simulink model "sampleModel354"  (R2021b)
settings: Solver=VariableStepAuto  StartTime=0.0  StopTime=10.0  RelTol=1e-3
libraries: simulink x2, slpidlib x1
settings Model: Creator=user  LastModifiedBy=user

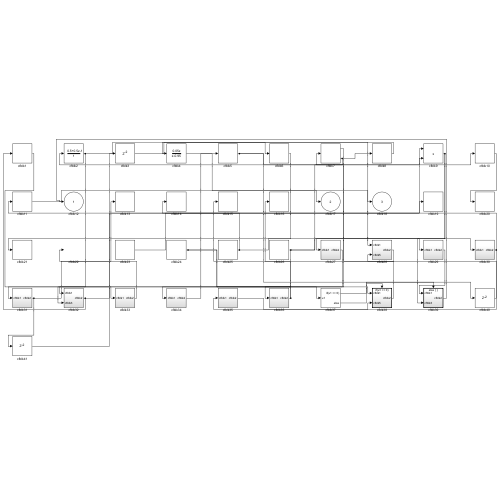
[thumbnail: Simulink's stored preview of the top-level diagram]
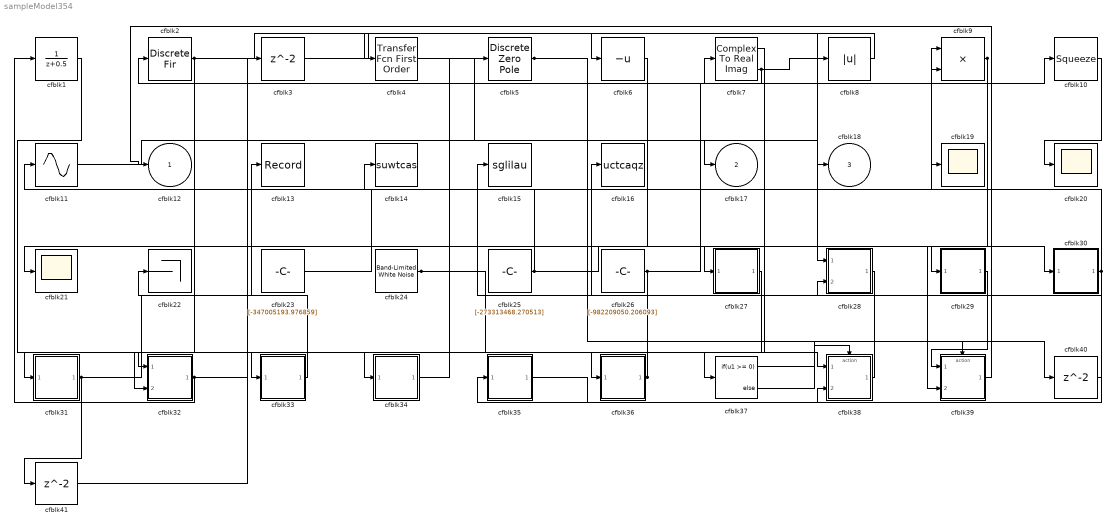
== system sampleModel354 ==
  cfblk1 : DiscreteTransferFcn  SampleTime=1
  cfblk10 : Squeeze
  cfblk11 : Sin  TimeSource=Use external signal  SampleTime=0
  cfblk13 : Record  FileSettingsInternal="{\"entries\":[{\"content\":{\"excelSettings\":{\"content\":{},\"type\":\"Streamout.ExcelSettings\"}},\"type\":\"Streamout.FileSettingStorage\",\"uuid\":\"651ccca9-41b0-448b-87a9-5c5838d69a5d\"}],\"packageUris\":[\"http://schema.mathworks.com/mf0/streamout_blocks/R2020a\"],\"version\":\"1.0\"}"  SignalsInternal="{\"entries\":[{\"content\":{\"signals\":[{\"content\":{\"blockPath\":[\"sampleModel354/cfblk13\"],\"channel\":[],\"dimensions\":[1],\"domain\":\"sampleModel354/cfblk13\",\"lineColor\":\"#b746ff\",\"plots\":[1],\"port\":1,\"sid\":[\"\"],\"signalID\":14731,\"signalName\":\"cfblk31\"},\"type\":\"RecordBlkView.Signal\",\"uuid\":\"0d68e5df-fecc-40d7-916a-77594ce0a885\"}]},\"type\":\"RecordBlkView.InputSignals\",\"uuid\":\"2bd33199-b1ec-44f2-9605-e6013ce188e2\"}],\"packageUris\":[\"http://schema.mathworks.com/mf0/streamout_blocks/R2020a\"],\"version\":\"1.0\"}"  VisualizationBindings="{\"sparklinesplugin\":{\"info\":[{\"bindingParametersList\":[],\"subplotID\":1}]}}"
  cfblk14 : ToWorkspace  VariableName=suwtcas  SaveFormat=Timeseries  SampleTime=-1
  cfblk15 : ToWorkspace  VariableName=sglilau  SaveFormat=Timeseries  SampleTime=-1
  cfblk16 : ToWorkspace  VariableName=uctcaqz  SaveFormat=Timeseries  SampleTime=-1
  cfblk19 : Scope
  cfblk2 : DiscreteFir  SampleTime=1
  cfblk20 : Scope
  cfblk21 : Scope
  cfblk22 : Terminator
  cfblk23 : Constant  Value=[-347005193.976859]  SampleTime=1
  cfblk24 : simulink/Sources/Band-Limited White Noise  Cov=[1107350414.755051]  Ts=0.1  seed=[9554781753.000000]
  cfblk25 : Constant  Value=[-273313468.270513]  SampleTime=1
  cfblk26 : Constant  Value=[-982209050.206093]  SampleTime=1
  cfblk27 : Subsystem
  cfblk28 : Subsystem
  cfblk29 : Subsystem
  cfblk3 : Delay  SampleTime=1
  cfblk30 : Subsystem
  cfblk31 : Subsystem
  cfblk32 : Subsystem
  cfblk33 : Subsystem
  cfblk34 : Subsystem
  cfblk35 : Subsystem
  cfblk36 : Subsystem
  cfblk37 : If  IfExpression=u1 >= 0  SampleTime=1
  cfblk38 : Subsystem  TreatAsAtomicUnit=on
  cfblk39 : Subsystem  TreatAsAtomicUnit=on
  cfblk4 : simulink/Discrete/Transfer Fcn First Order  PoleZ=0.95  ICPrevOutput=0.0  DoSatur=off
  cfblk40 : Delay  SampleTime=1
  cfblk41 : Delay  SampleTime=1
  cfblk5 : DiscreteZeroPole  Poles=[0 0.5]  Gain=1
  cfblk6 : UnaryMinus
  cfblk7 : ComplexToRealImag
  cfblk8 : Abs
  cfblk9 : Product
  cfblk12 : Outport
  cfblk17 : Outport  Port=2
  cfblk18 : Outport  Port=3
  wires:
  cfblk34/1(cfblk2) -> cfblk5/1
  cfblk3/1 -> cfblk28/1(cfblk1)
  cfblk27/1(cfblk2) -> cfblk36/1(cfblk1)
  cfblk28/1(cfblk2) -> cfblk7/1
  cfblk6/1 -> cfblk21/1
  cfblk29/1(cfblk2) -> cfblk39/1(cfblk1)
  cfblk1/1 -> cfblk33/1(cfblk1)
  cfblk38/1(cfblk2) -> cfblk16/1
  cfblk5/1 -> cfblk9/2, cfblk40/1
  cfblk9/1 -> cfblk27/1(cfblk1), cfblk39/2(cfblk3)
  cfblk7/1 -> cfblk34/1(cfblk1)
  cfblk10/1 -> cfblk20/1
  cfblk7/2 -> cfblk2/1, cfblk8/1
  cfblk33/1(cfblk2) -> cfblk22/1
  cfblk4/1 -> cfblk17/1
  cfblk24/1 -> cfblk38/1(cfblk1), cfblk37/1
  cfblk30/1(cfblk2) -> cfblk35/1(cfblk1), cfblk14/1
  cfblk2/1 -> cfblk6/1, cfblk32/1(cfblk1)
  cfblk11/1 -> cfblk18/1
  cfblk39/1(cfblk2) -> cfblk12/1
  cfblk23/1 -> cfblk9/1
  cfblk36/1(cfblk2) -> cfblk15/1, cfblk31/1(cfblk1)
  cfblk31/1(cfblk2) -> cfblk13/1, cfblk41/1
  cfblk8/1 -> cfblk4/1
  cfblk25/1 -> cfblk11/1, cfblk29/1(cfblk1)
  cfblk26/1 -> cfblk10/1, cfblk32/2(cfblk3), cfblk30/1(cfblk1)
  cfblk35/1(cfblk2) -> cfblk38/2(cfblk5)
  cfblk32/1(cfblk2) -> cfblk1/1, cfblk19/1
  cfblk37/1 -> cfblk38/Action
  cfblk37/2 -> cfblk39/Action
  cfblk40/1 -> cfblk28/2(cfblk5)
  cfblk41/1 -> cfblk3/1

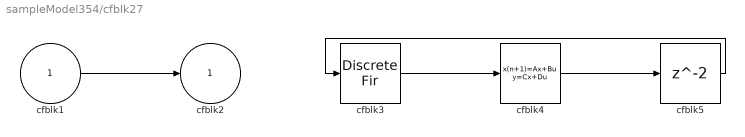
== system sampleModel354/cfblk27 ==
  cfblk1 : Inport
  cfblk3 : DiscreteFir  SampleTime=1
  cfblk4 : DiscreteStateSpace
  cfblk5 : Delay  SampleTime=1
  cfblk2 : Outport
  wires:
  cfblk1/1 -> cfblk2/1
  cfblk3/1 -> cfblk4/1
  cfblk4/1 -> cfblk5/1
  cfblk5/1 -> cfblk3/1

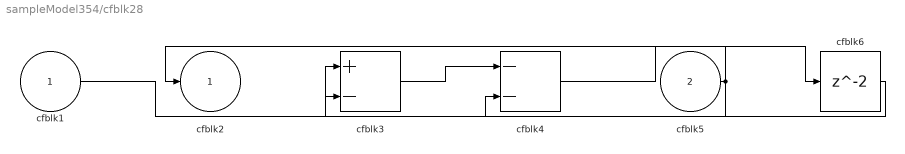
== system sampleModel354/cfblk28 ==
  cfblk1 : Inport
  cfblk5 : Inport  Port=2
  cfblk3 : Sum  Inputs=+-
  cfblk4 : Sum  Inputs=--
  cfblk6 : Delay  SampleTime=1
  cfblk2 : Outport
  wires:
  cfblk5/1 -> cfblk2/1, cfblk4/2
  cfblk1/1 -> cfblk3/1
  cfblk3/1 -> cfblk4/1
  cfblk4/1 -> cfblk6/1
  cfblk6/1 -> cfblk3/2

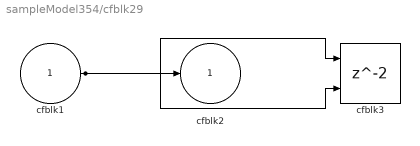
== system sampleModel354/cfblk29 ==
  cfblk1 : Inport
  cfblk3 : Delay  ShowEnablePort=on  SampleTime=1
      settings: InputPortMap=u0,e6
  cfblk2 : Outport
  wires:
  cfblk1/1 -> cfblk2/1, cfblk3/1, cfblk3/2

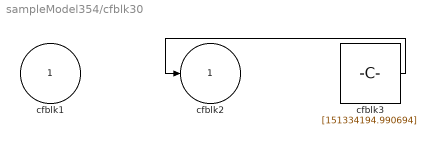
== system sampleModel354/cfblk30 ==
  cfblk1 : Inport
  cfblk3 : Constant  Value=[151334194.990694]  SampleTime=1
  cfblk2 : Outport
  wires:
  cfblk3/1 -> cfblk2/1

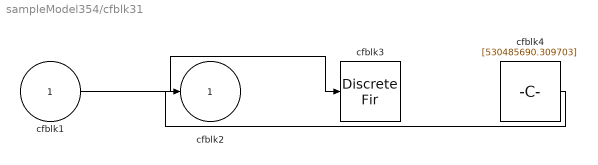
== system sampleModel354/cfblk31 ==
  cfblk1 : Inport
  cfblk3 : DiscreteFir  SampleTime=1
  cfblk4 : Constant  Value=[530485690.309703]  SampleTime=1
  cfblk2 : Outport
  wires:
  cfblk1/1 -> cfblk3/1
  cfblk4/1 -> cfblk2/1

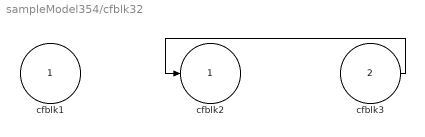
== system sampleModel354/cfblk32 ==
  cfblk1 : Inport
  cfblk3 : Inport  Port=2
  cfblk2 : Outport
  wires:
  cfblk3/1 -> cfblk2/1

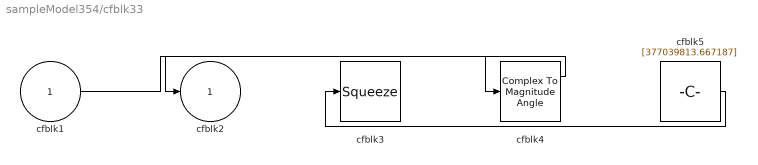
== system sampleModel354/cfblk33 ==
  cfblk1 : Inport
  cfblk3 : Squeeze
  cfblk4 : ComplexToMagnitudeAngle
  cfblk5 : Constant  Value=[377039813.667187]  SampleTime=1
  cfblk2 : Outport
  wires:
  cfblk4/1 -> cfblk2/1
  cfblk5/1 -> cfblk3/1
  cfblk1/1 -> cfblk4/1

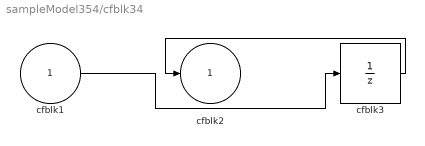
== system sampleModel354/cfblk34 ==
  cfblk1 : Inport
  cfblk3 : UnitDelay  HasFrameUpgradeWarning=on
  cfblk2 : Outport
  wires:
  cfblk3/1 -> cfblk2/1
  cfblk1/1 -> cfblk3/1

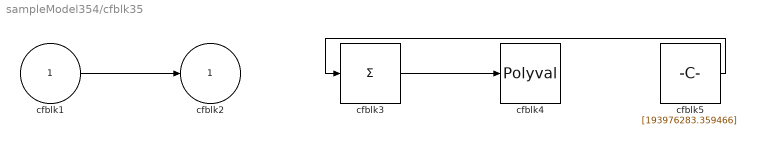
== system sampleModel354/cfblk35 ==
  cfblk1 : Inport
  cfblk3 : Sum  Inputs=+
  cfblk4 : Polyval  Coefs=[ +2.081618890e-019, -1.441693666e-014, +4.719686976e-010, -8.536869453e-006, +1.621573104e-001, -8.087801117e+001 ]
  cfblk5 : Constant  Value=[193976283.359466]  SampleTime=1
  cfblk2 : Outport
  wires:
  cfblk3/1 -> cfblk4/1
  cfblk5/1 -> cfblk3/1
  cfblk1/1 -> cfblk2/1

== system sampleModel354/cfblk36 ==
  cfblk1 : Inport
  cfblk3 : slpidlib/PID Controller  Controller=PID  Form=Parallel  TimeDomain=Discrete-time  UseExternalTs=off  SampleTime=1  IntegratorMethod=Forward Euler  FilterMethod=Forward Euler  ControllerParametersSource=internal  P=1  I=1  D=0  UseFilter=on  N=100  TunerSelectOption=Transfer Function Based (PID Tuner App)  InitialConditionSource=internal  InitialConditionForIntegrator=0  InitialConditionForFilter=0  DifferentiatorICPrevScaledInput=0  ExternalReset=none  TrackingMode=off  Kt=1  LimitOutput=off  SatLimitsSource=internal  UpperSaturationLimit=inf  LowerSaturationLimit=-inf  LinearizeAsGain=off  AntiWindupMode=none  Kb=1  POutMin=[]  POutMax=[]  IOutMin=[]  IOutMax=[]  DOutMin=[]  DOutMax=[]  NOutMin=[]  NOutMax=[]  SumOutMin=[]  SumOutMax=[]  SaturationOutMin=[]  SaturationOutMax=[]  PParamMin=[]  PParamMax=[]  IParamMin=[]  IParamMax=[]  DParamMin=[]  DParamMax=[]  NParamMin=[]  NParamMax=[]  KbParamMin=[]  KbParamMax=[]  KtParamMin=[]  KtParamMax=[]  KbOutMin=[]  KbOutMax=[]  KtOutMin=[]  KtOutMax=[]  IntegratorOutMin=[]  IntegratorOutMax=[]  FilterOutMin=[]  FilterOutMax=[]  SumI1OutMin=[]  SumI1OutMax=[]  SumI2OutMin=[]  SumI2OutMax=[]  SumI3OutMin=[]  SumI3OutMax=[]  SumI4OutMin=[]  SumI4OutMax=[]  SumDOutMin=[]  SumDOutMax=[]  DifferentiatorOutMin=[]  DifferentiatorOutMax=[]  FilterDiffOutCoefMin=[]  FilterDiffOutCoefMax=[]  ReciprocalOutMin=[]  ReciprocalOutMax=[]  SumDenOutMin=[]  SumDenOutMax=[]  SumNumOutMin=[]  SumNumOutMax=[]  DivideOutMin=[]  DivideOutMax=[]  UdiffTsProdOutMin=[]  UdiffTsProdOutMax=[]  NTsProdOutMin=[]  NTsProdOutMax=[]  UintegralTsProdOutMin=[]  UintegralTsProdOutMax=[]  UngainTsProdOutMin=[]  UngainTsProdOutMax=[]  IntegratorContinuousStateAttributes=''  IntegratorStateMustResolveToSignalObject=off  IntegratorRTWStateStorageClass=Auto  FilterContinuousStateAttributes=''  FilterStateMustResolveToSignalObject=off  FilterRTWStateStorageClass=Auto  ParallelPVariant=InternalParameters  IdealPVariant=Disabled  IVariant=InternalParameters  DVariant=InternalParameters  IntegratorVariant=Discrete  SatVariant=Disabled  AWVariant=Passthrough  PCopyVariant=Disabled  TRVariant=Disabled  FdbkBlocksVariant=Forward  IdealPFdbkVariant=Disabled  SatFdbkVariant=Disabled  DerivativeFilterVariant=ForwardEulerFilter  NVariant=InternalParameters  NCopyVariant=Disabled  FilterICVariant=InternalICsFilter  IntegratorICVariant=InternalICs  ExternalResetVariant=Disabled  TRSumVariant=Passthrough  SumFdbkVariant=Disabled  SumVariant=Sum_PID  TsampFilterVariant=InternalTs  TsampNgainVariant=Passthrough  TsampIntegralVariant=Passthrough  ExternalSaturationOutDataTypeStr=Inherit: Same as second input
  cfblk2 : Outport
  wires:
  cfblk3/1 -> cfblk2/1
  cfblk1/1 -> cfblk3/1

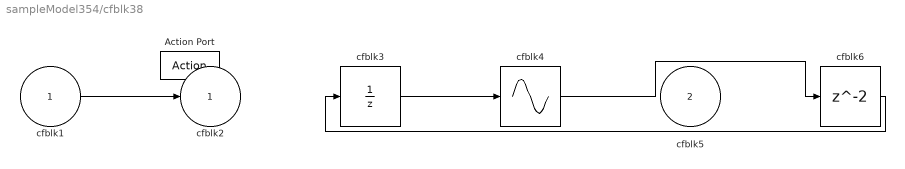
== system sampleModel354/cfblk38 ==
  cfblk1 : Inport
  cfblk5 : Inport  Port=2
  Action Port : ActionPort  ActionPortLabel=if(u1 >= 0)
  cfblk3 : UnitDelay  SampleTime=-1  HasFrameUpgradeWarning=on
  cfblk4 : Sin  TimeSource=Use external signal  SampleTime=0
  cfblk6 : Delay
  cfblk2 : Outport
  wires:
  cfblk1/1 -> cfblk2/1
  cfblk3/1 -> cfblk4/1
  cfblk4/1 -> cfblk6/1
  cfblk6/1 -> cfblk3/1

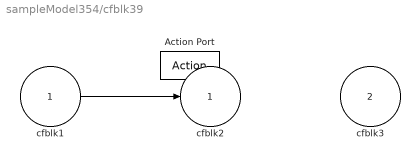
== system sampleModel354/cfblk39 ==
  cfblk1 : Inport
  cfblk3 : Inport  Port=2
  Action Port : ActionPort  ActionPortLabel=else
  cfblk2 : Outport
  wires:
  cfblk1/1 -> cfblk2/1
